simulink model "sistema_tipo_zero_degrau"  (R2017b)
settings: Solver=VariableStepAuto  StartTime=0.0  StopTime=3.0  RelTol=1e-3
settings Model: Creator=fernandopassold  LastModifiedBy=fernandopassold
settings CodeAppCC: StateflowObjectComments=on

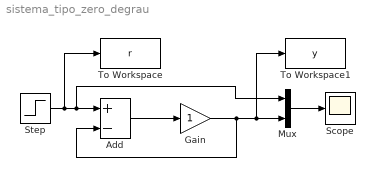
== system sistema_tipo_zero_degrau ==
  Add : Sum  Inputs=+-
  Gain : Gain
  Mux : Mux  Inputs=2
  Scope : Scope
  Step : Step  SampleTime=0
  To Workspace : ToWorkspace  VariableName=r  SaveFormat=Timeseries  SampleTime=-1
  To Workspace1 : ToWorkspace  VariableName=y  SaveFormat=Timeseries  SampleTime=-1
  wires:
  Add/1 -> Gain/1
  Step/1 -> To Workspace/1, Mux/1, Add/1
  Gain/1 -> Add/2, To Workspace1/1, Mux/2
  Mux/1 -> Scope/1
